simulink model "GK_model"  (Simulink 3.00)
settings: Solver=ode45  StartTime=0.0  StopTime=20  RelTol=1e-3
settings Model: Creator=angel  LastModifiedBy=angel

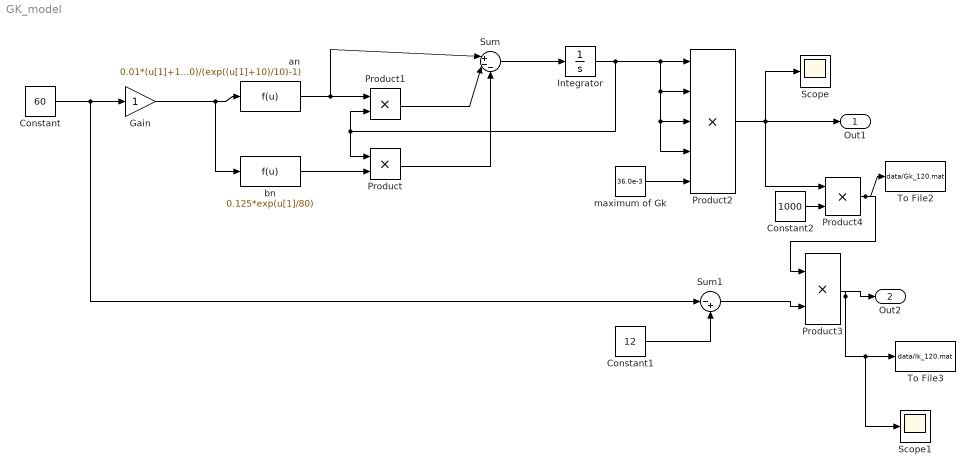
== system GK_model ==
  Constant : Constant  Value=60
  Constant1 : Constant  Value=12
  Constant2 : Constant  Value=1000
  Gain : Gain  Gain=1  SaturateOnIntegerOverflow=on
  Integrator : Integrator  ExternalReset=none  InitialConditionSource=internal  InitialCondition=0.31769  LimitOutput=off  UpperSaturationLimit=inf  LowerSaturationLimit=-inf  ShowSaturationPort=off  ShowStatePort=off  AbsoluteTolerance=auto
  Product{,1,3..4} (4 alike) : Product  Inputs=2  SaturateOnIntegerOverflow=on
  Product2 : Product  Inputs=5  SaturateOnIntegerOverflow=on
  Scope : Scope
      settings: TimeRange=20  YMin=0  YMax=0.04  SaveToWorkspace=off  SaveName=ScopeData
  Scope1 : Scope
      settings: TimeRange=20  YMin=0  YMax=0.04  SaveToWorkspace=off  SaveName=ScopeData
  Sum : Sum  Inputs=|+--  SaturateOnIntegerOverflow=on
  Sum1 : Sum  Inputs=|-+  SaturateOnIntegerOverflow=on
  To File2 : ToFile  Filename=data/Gk_120.mat  MatrixName=Gk  SampleTime=-1
  To File3 : ToFile  Filename=data/Ik_120.mat  MatrixName=Ik  SampleTime=-1
  an : Fcn  Expr=0.01*(u[1]+10)/(exp((u[1]+10)/10)-1)
  bn : Fcn  Expr=0.125*exp(u[1]/80)
  maximum of Gk : Constant  Value=36.0e-3
  Out1 : Outport  Port=1
  Out2 : Outport  Port=2
  wires:
  bn/1 -> Product/2
  an/1 -> Product1/1, Sum/1
  Product1/1 -> Sum/2
  Product/1 -> Sum/3
  Sum/1 -> Integrator/1
  Integrator/1 -> Product1/2, Product/1, Product2/1, Product2/2, Product2/3, Product2/4
  maximum of Gk/1 -> Product2/5
  Gain/1 -> an/1, bn/1
  Product2/1 -> Scope/1, Out1/1, Product4/1
  Constant/1 -> Gain/1, Sum1/1
  Constant1/1 -> Sum1/2
  Sum1/1 -> Product3/2
  Product3/1 -> Out2/1, To File3/1, Scope1/1
  Constant2/1 -> Product4/2
  Product4/1 -> To File2/1, Product3/1
